simulink model "Praktikum11Gruppe09"  (R2023b)
settings: Solver=VariableStepAuto  StartTime=0.0  StopTime=0.05  RelTol=1e-3
model workspace (MAT data in the model file):
  CodeRate = 0.75
  M = 16
  PunctureVector = [1; 1; 0; 1; 0; 1]
  TracebackDepth = 48
  Trelli.numInputSymbols = 2
  Trelli.numOutputSymbols = 4
  Trelli.numStates = 64
  Trelli.nextStates = [0  32; 0  32; 1  33; 1  33; 2  34; 2  34; 3  35; 3  35; 4  36; 4  36; 5  37; 5  37; 6  38; 6  38; 7  39; 7  39; 8  40; 8  40; 9  41; 9  41; 10  42; 10  42; 11  43; 11  43; 12  44; 12  44; 13  45; 13  45; 14  46; 14  46; 15  47; 15  47; 16  48; 16  48; 17  49; 17  49; 18  50; 18  50; 19  51; 19  51; 20  52; 20  52; 21  53; 21  53; 22  54; 22  54; 23  55; 23  55; 24  56; 24  56; 25  57; 25  57; 26  58; 26  58; 27  59; 27  59; 28  60; 28  60; 29  61; 29  61; 30  62; 30  62; 31  63; 31  63]
  Trelli.outputs = [0  3; 3  0; 1  2; 2  1; 0  3; 3  0; 1  2; 2  1; 3  0; 0  3; 2  1; 1  2; 3  0; 0  3; 2  1; 1  2; 3  0; 0  3; 2  1; 1  2; 3  0; 0  3; 2  1; 1  2; 0  3; 3  0; 1  2; 2  1; 0  3; 3  0; 1  2; 2  1; 2  1; 1  2; 3  0; 0  3; 2  1; 1  2; 3  0; 0  3; 1  2; 2  1; 0  3; 3  0; 1  2; 2  1; 0  3; 3  0; 1  2; 2  1; 0  3; 3  0; 1  2; 2  1; 0  3; 3  0; 2  1; 1  2; 3  0; 0  3; 2  1; 1  2; 3  0; 0  3]
  Ts = 5e-08
undefined symbols (not defined in the file): doppler, get, gray, hot, j, magnitude
libraries: dspxfrm3 x6, dspstat3 x5, dspsigops x5, dspobslib x4, commrflib2 x3, commcnvcod2 x3, commdigbbndam3 x3, dspindex x3, commchan3 x2, commrandsrc3 x2, dspquant2 x2, commsink2 x2
settings Model: Creator=suttarar@hu-berlin.de  LastModifiedBy=suttarar@hu-berlin.de

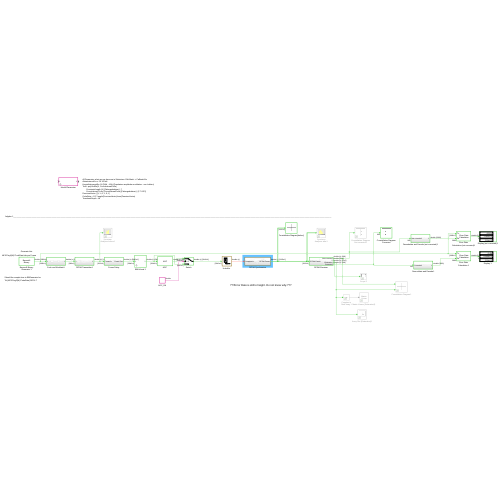
[thumbnail: Simulink's stored preview of the top-level diagram]
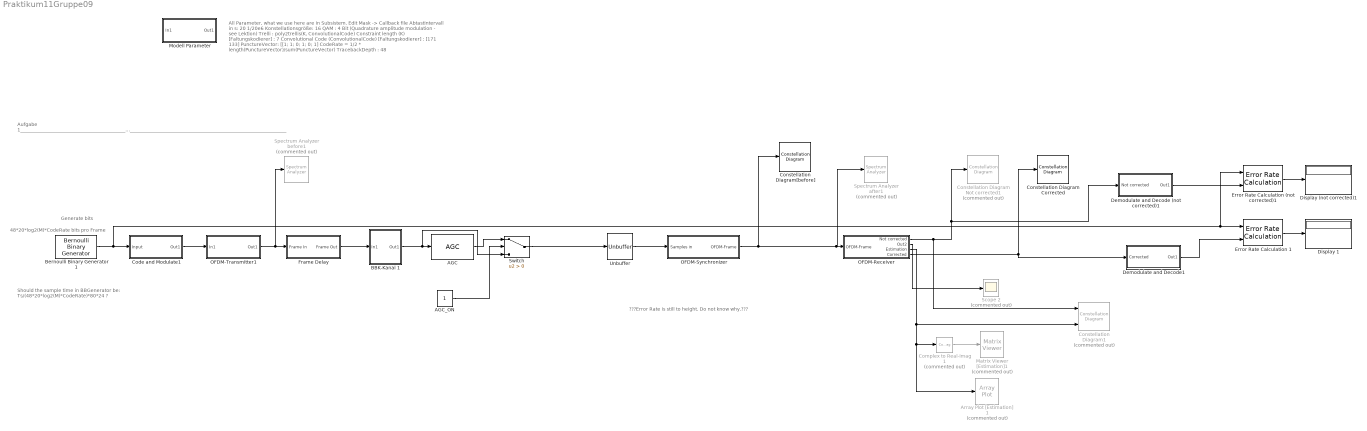
== system Praktikum11Gruppe09 ==
  note: ???Error Rate is still to height. Do not know why.???
  note: Aufgabe 1______________________________________________________________________________________________________________________________________________________________________________________________________________________________________________________________________________________________________________
  note: Should the sample time in BBGenerator be:
      | Ts/(48*20*log2(M)*CodeRate)*80*24 ?
  note: All Parameter, what we use here are in Subsistem. Edit Mask -> Callback file
      | Abtastintervall in s: 20 1/20e6
      | Konstellationsgröße: 16 QAM : 4 Bit (Quadrature amplitude modulation - see Lektion)
      | Trelli : poly2trellis(K, ConvolutionalCode)
      | Constraint length (K) [Faltungskodierer] : 7
      | Convolutional Code (ConvolutionalCode) [Faltungskodierer] : [171 133]
      | PunctureVector: [[1; 1; 0; 1; 0; 1]
      | CodeRate = 1/2 * length(PunctureVector)/sum(PunctureVector)
      | TracebackDepth : 48
  note: 48*20*log2(M)*CodeRate bits pro Frame
  note: Generate bits
  "AGC " : commrfcorlib/AGC  LegacyMode=off  DetectorMethod=Rectifier  LoopMethod=Linear  UpdatePeriod=100  StepSize=0.1  AdaptationStepSize=0.01  DesiredOutputPower=1  AveragingLength=16  MaximumGain=30  MaxPowerGain=10  GainOutputPort=off  InputPowerOutputPort=off  SimulateUsing=Interpreted execution
  AGC_ON : Constant
  Array Plot [Estimation]1 : ArrayPlot  Commented=on  WindowPosition=[886.000000,184.000000,800.000000,500.000000,]  ScopeFrameLocation=window  PlotAsMagnitudePhase=on  YLimits=[-0.4803 1.494]
  BBK-Kanal 1 : Subsystem  mask{MaxDoppler=20, PathDelays=[0 2 5].*Ts, PathGains=[0 -16 -24], EnableMultipath=1, PathLoss=0, FrequencyOffset=50000, PhaseOffset=0, SNR=25}
      mask prompts: MaxDoppler "Dopplerverschiebung"; PathDelays "Pfadverzoergerungen"; PathGains "Pfadverstaerkungen"; EnableMultipath "SwitchBlock"; PathLoss "Pfadverlust"; FrequencyOffset "Frequenzverschiebung"; PhaseOffset "Phasenverschiebung"; SNR "AWG-Rauschen"
  Bernoulli Binary Generator 1 : commrandsrc3/Bernoulli Binary Generator  ProbabilityOfZero=0.5  SeedSource=Auto  Seed=0  SampleTime=Ts/(48*20*log2(M)*CodeRate)*80*24  SamplesPerFrame=48*20*log2(M)*CodeRate  OutputDataType=double  SimulateUsing=Interpreted execution
  Code and Modulate1 : Subsystem
  Complex to Real-Imag 1 : ComplexToRealImag  Commented=on  Output=Real
  Constellation Diagram Corrected : ConstellationDiagram  WindowPosition=[869.000000,188.000000,600.000000,600.000000,]  ScopeFrameLocation=window  SymbolsToDisplaySource=Property  SymbolsToDisplay=500  ReferenceConstellation="[0.70711+0.70711i        -0.70711+0.70711i        -0.70711-0.70711i         0.70711-0.70711i]"  XLimits=[-1.71,1.66]  YLimits=[-1.67,1.51]  ShowLegend=on
  Constellation Diagram Not corrected1 : ConstellationDiagram  Commented=on  WindowPosition=[922.000000,306.000000,600.000000,600.000000,]  ScopeFrameLocation=window  ReferenceConstellation="[0.70711+0.70711i        -0.70711+0.70711i        -0.70711-0.70711i         0.70711-0.70711i]"  XLimits=[-1.55,1.51]  YLimits=[-1.43,1.46]  ShowLegend=on
  Constellation Diagram1 : ConstellationDiagram  Commented=on  NumInputPorts=2  WindowPosition=[1234.000000,143.000000,600.000000,600.000000,]  ScopeFrameLocation=window  ReferenceConstellation="{[0.70711+0.70711i        -0.70711+0.70711i        -0.70711-0.70711i         0.70711-0.70711i][0.70711+0.70711i        -0.70711+0.70711i        -0.70711-0.70711i         0.70711-0.70711i]}"  XLimits=[-1.55,1.51]  YLimits=[-1.43,1.46]  ShowLegend=on
  Constellation Diagram[before] : ConstellationDiagram  WindowPosition=[219.000000,183.000000,600.000000,600.000000,]  ScopeFrameLocation=window  SymbolsToDisplaySource=Property  SymbolsToDisplay=500  ReferenceConstellation="[0.70711+0.70711i        -0.70711+0.70711i        -0.70711-0.70711i         0.70711-0.70711i]"  XLimits=[-1.71,1.66]  YLimits=[-1.67,1.51]  ShowLegend=on
  Demodulate and Decode (not corrected)1 : Subsystem
  Demodulate and Decode1 : Subsystem
  Display (not corrected)1 : Display
  Display 1 : Display
  Error Rate Calculation (not corrected)1 : commsink2/Error Rate Calculation  N=TracebackDepth  st_delay=48*20*log2(M)*CodeRate  cp_mode=Entire frame  subframe=[]  PMode=Port  WsName=ErrorVec  RsMode2=off  stop=off  numErr=100  maxBits=1e6
  Error Rate Calculation 1 : commsink2/Error Rate Calculation  N=TracebackDepth+2880  st_delay=0  cp_mode=Entire frame  subframe=[]  PMode=Port  WsName=ErrorVec  RsMode2=off  stop=off  numErr=100  maxBits=1e6
  Frame Delay : Subsystem
  Matrix Viewer [Estimation]1 : dspobslib/Matrix Viewer  Commented=on  ImageParams=off  CMapStr=gray(256)  AxisColorbar=on  AxisParams=off  AxisOrigin=Upper left corner  AxisTickMode=Auto  XTickRange=[0 1]  YTickRange=[0 1]  XLabel=X-axis  YLabel=Y-axis  ZLabel=Z-axis  FigPos=get(0,'defaultfigureposition')  AxisZoom=off
      settings: YMin=0.99546  YMax=1.0044
  Modell Parameter : Subsystem  mask{Ts=1/20e6, M=16, Trelli=poly2trellis(7, [171 133]), PunctureVector=[1; 1; 0; 1; 0; 1], CodeRate=0.75, TracebackDepth=48}
      mask prompts: Ts "Abtastintervall in s"; M "Konstellationsgröße"
  "OFDM-Receiver " : Subsystem
  OFDM-Synchronizer : Subsystem
  OFDM-Transmitter1 : Subsystem
  Scope 2 : Scope  Commented=on
  Spectrum Analyzer after1 : SpectrumAnalyzer  Commented=on  WindowPosition=[940.000000,172.000000,800.000000,500.000000,]  Visible=on  ScopeFrameLocation=window  Span=20000000  StartFrequency=-10000000  StopFrequency=10000000  YLimits=[-28.40563685,17.66109951]
  Spectrum Analyzer before1 : SpectrumAnalyzer  Commented=on  WindowPosition=[6.000000,502.000000,800.000000,500.000000,]  ScopeFrameLocation=window  Span=20000000  StartFrequency=-10000000  StopFrequency=10000000  YLimits=[-48.78355479,20.07673212]
  "Switch " : Switch  Criteria=u2 > Threshold  SaturateOnIntegerOverflow=off  InputSameDT=off
  "Unbuffer " : Unbuffer
  wires:
  "OFDM-Receiver "/1(Not corrected) -> Constellation Diagram1/1, Demodulate and Decode (not corrected)1/1(Not corrected), Constellation Diagram Not corrected1/1
  Code and Modulate1/1(Out1) -> OFDM-Transmitter1/1(In1)
  Complex to Real-Imag 1/1 -> Matrix Viewer [Estimation]1/1
  "OFDM-Receiver "/2(Out2) -> Scope 2/1
  "OFDM-Receiver "/4(Corrected) -> Demodulate and Decode1/1(Corrected), Constellation Diagram Corrected/1
  Error Rate Calculation 1/1 -> Display 1/1
  Error Rate Calculation (not corrected)1/1 -> Display (not corrected)1/1
  Demodulate and Decode (not corrected)1/1(Out1) -> Error Rate Calculation (not corrected)1/2
  OFDM-Transmitter1/1(Out1) -> Spectrum Analyzer before1/1, Frame Delay/1(Frame In)
  Demodulate and Decode1/1(Out1) -> Error Rate Calculation 1/2
  Bernoulli Binary Generator 1/1 -> Error Rate Calculation (not corrected)1/1, Error Rate Calculation 1/1, Code and Modulate1/1(Input)
  "OFDM-Receiver "/3(Estimation) -> Constellation Diagram1/2, Array Plot [Estimation]1/1, Complex to Real-Imag 1/1
  "Unbuffer "/1 -> OFDM-Synchronizer/1(Samples in)
  BBK-Kanal 1/1(Out1) -> "Switch "/3, "AGC "/1
  Frame Delay/1(Frame Out) -> BBK-Kanal 1/1(In1)
  "Switch "/1 -> "Unbuffer "/1
  "AGC "/1 -> "Switch "/1
  AGC_ON/1 -> "Switch "/2
  OFDM-Synchronizer/1(OFDM-Frame) -> Spectrum Analyzer after1/1, "OFDM-Receiver "/1(OFDM-Frame), Constellation Diagram[before]/1

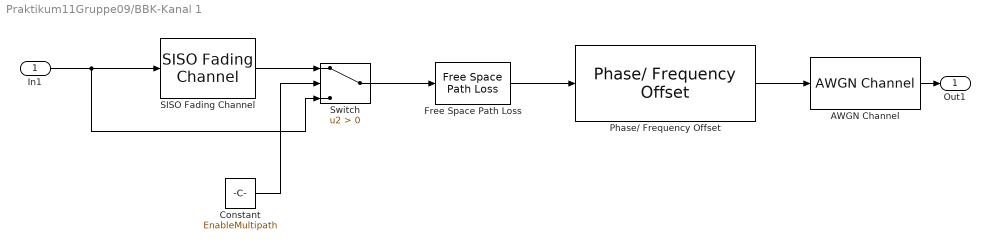
== system Praktikum11Gruppe09/BBK-Kanal 1 ==
  In1 : Inport
  AWGN Channel : commchan3/AWGN Channel  LegacyMode=off  NoiseMethod="Signal to noise ratio  (SNR)"  noiseMode="Signal to noise ratio  (SNR)"  EbNo=10  EsNo=10  SNR=SNR  BitsPerSymbol=1  SignalPower=1  SamplesPerSymbol=1  SymbolPeriod=1  VarianceSource=Parameter  Variance=1  RandomStream=Global stream  Seed=67  SimulateUsing=Code generation
  Constant : Constant  Value=EnableMultipath
  Free Space Path Loss : commrflib2/Free Space Path Loss  mode=Decibels  dB=PathLoss  d=0.100  fc=1920
  Phase/ Frequency Offset : commrflib2/Phase// Frequency Offset  phaseOffset=PhaseOffset  freqPort=off  freqOffset=FrequencyOffset
      settings: LibrarySourceBlock=|
      | commrfcorlib/Phase//
      | Frequency
      | Offset
  SISO Fading Channel : commchan3/SISO Fading Channel  InheritSampleRate=on  SampleRate=1  PathDelays=PathDelays  AveragePathGains=PathGains  NormalizePathGains=on  FadingDistribution=Rayleigh  KFactor=3  DirectPathDopplerShift=0  DirectPathInitialPhase=0  MaximumDopplerShift=MaxDoppler  DopplerSpectrum=doppler('Jakes')  RandomStream=mt19937ar with seed  Seed=73  PathGainsOutputPort=off  ChannelFilterDelayOutputPort=off  SimulateUsing=Interpreted execution  Visualization=Off  PathsForDopplerDisplay=1  SamplesToDisplay=25%
  Switch : Switch  Criteria=u2 > Threshold  SaturateOnIntegerOverflow=off  InputSameDT=off
  Out1 : Outport
  wires:
  Phase/ Frequency Offset/1 -> AWGN Channel/1
  Free Space Path Loss/1 -> Phase/ Frequency Offset/1
  AWGN Channel/1 -> Out1/1
  Switch/1 -> Free Space Path Loss/1
  SISO Fading Channel/1 -> Switch/1
  In1/1 -> Switch/3, SISO Fading Channel/1
  Constant/1 -> Switch/2

== system Praktikum11Gruppe09/Code and Modulate1 ==
  note: Modulation
  note: Faltungscodierer
  Input : Inport
  "Convolutional Encoder " : commcnvcod2/Convolutional Encoder  trellis=Trelli  opMode=Continuous  DelayedResetAction=off  hasIniStPort=off  hasFinStPort=off  usePuncVector=on  punctureVector=PunctureVector  reset=Unused parameter value
  "Rectangular QAM Modulator Baseband " : commdigbbndam3/Rectangular QAM Modulator Baseband  M=M  InType=Bit  Enc=Gray  Mapping=[0:15]  PowType=Average Power  MinDist=2  AvgPow=1  PeakPow=1  Ph=0  outDtype=double  outWordLen=16  outUDDataType=sfix(16)  outFracLenMode=Best precision  outFracLen=15  outDataTypeStr=double  outLastDataTypeStr=double
  Out1 : Outport
  wires:
  "Convolutional Encoder "/1 -> "Rectangular QAM Modulator Baseband "/1
  "Rectangular QAM Modulator Baseband "/1 -> Out1/1
  Input/1 -> "Convolutional Encoder "/1

== system Praktikum11Gruppe09/Demodulate and Decode (not corrected)1 ==
  Not corrected : Inport
  "Data Type Conversion " : DataTypeConversion  SaturateOnIntegerOverflow=off  RndMeth=Floor
  "Gain " : Gain  Gain=-1
  "Rectangular QAM Demodulator Baseband " : commdigbbndam3/Rectangular QAM Demodulator Baseband  M=M  OutType=Bit  DecType=Approximate log-likelihood ratio  VarSource=Dialog  Variance=1  Dec=Gray  Mapping=[0:15]  PowType=Average Power  MinDist=2  AvgPow=1  PeakPow=1  Ph=0  outDtype1=Inherit via internal rule  outDtype2=Inherit via internal rule  derotateFactorWordLen=16  derotateFactorDataTypeStr=Inherit: Same word length as input  derotateFactorLastDataTypeStr=Inherit: Same word length as input  denormFactorWordLen=16  denormFactorDataTypeStr=Inherit: Same word length as input  denormFactorLastDataTypeStr=Inherit: Same word length as input  prodOutWordLen=32  prodOutOverflowMode=Wrap  prodOutRoundingMode=Floor  prodOutOvFlMode=off  prodOutOvFlModeLastStrValue=off  sumWordLen=32
  "Uniform Encoder " : dspquant2/Uniform Encoder  peak=1  bits=4  otype=Unsigned integer
  "Viterbi Decoder " : commcnvcod2/Viterbi Decoder  trellis=Trelli  isPunctured=on  punctureVector=PunctureVector  erasures=off  dectype=Soft decision  nsdecb=4  runSigValErrCheck=off  tbdepth=TracebackDepth  opmode=Continuous  reset=off  delayedResetAction=off  smWordLength=16  outDataType=double
  Out1 : Outport
  wires:
  "Uniform Encoder "/1 -> "Data Type Conversion "/1
  "Gain "/1 -> "Uniform Encoder "/1
  "Data Type Conversion "/1 -> "Viterbi Decoder "/1
  "Rectangular QAM Demodulator Baseband "/1 -> "Gain "/1
  Not corrected/1 -> "Rectangular QAM Demodulator Baseband "/1
  "Viterbi Decoder "/1 -> Out1/1

== system Praktikum11Gruppe09/Demodulate and Decode1 ==
  Corrected : Inport
  "Data Type Conversion " : DataTypeConversion  SaturateOnIntegerOverflow=off  RndMeth=Floor
  "Gain " : Gain  Gain=-1
  "Rectangular QAM Demodulator Baseband " : commdigbbndam3/Rectangular QAM Demodulator Baseband  M=M  OutType=Bit  DecType=Approximate log-likelihood ratio  VarSource=Dialog  Variance=1  Dec=Gray  Mapping=[0:15]  PowType=Average Power  MinDist=2  AvgPow=1  PeakPow=1  Ph=0  outDtype1=Inherit via internal rule  outDtype2=Inherit via internal rule  derotateFactorWordLen=16  derotateFactorDataTypeStr=Inherit: Same word length as input  derotateFactorLastDataTypeStr=Inherit: Same word length as input  denormFactorWordLen=16  denormFactorDataTypeStr=Inherit: Same word length as input  denormFactorLastDataTypeStr=Inherit: Same word length as input  prodOutWordLen=32  prodOutOverflowMode=Wrap  prodOutRoundingMode=Floor  prodOutOvFlMode=off  prodOutOvFlModeLastStrValue=off  sumWordLen=32
  "Uniform Encoder " : dspquant2/Uniform Encoder  peak=1  bits=4  otype=Unsigned integer
  "Viterbi Decoder " : commcnvcod2/Viterbi Decoder  trellis=Trelli  isPunctured=on  punctureVector=PunctureVector  erasures=off  dectype=Soft decision  nsdecb=4  runSigValErrCheck=off  tbdepth=TracebackDepth  opmode=Continuous  reset=off  delayedResetAction=off  smWordLength=16  outDataType=double
  Out1 : Outport
  wires:
  "Uniform Encoder "/1 -> "Data Type Conversion "/1
  "Gain "/1 -> "Uniform Encoder "/1
  "Data Type Conversion "/1 -> "Viterbi Decoder "/1
  "Rectangular QAM Demodulator Baseband "/1 -> "Gain "/1
  Corrected/1 -> "Rectangular QAM Demodulator Baseband "/1
  "Viterbi Decoder "/1 -> Out1/1

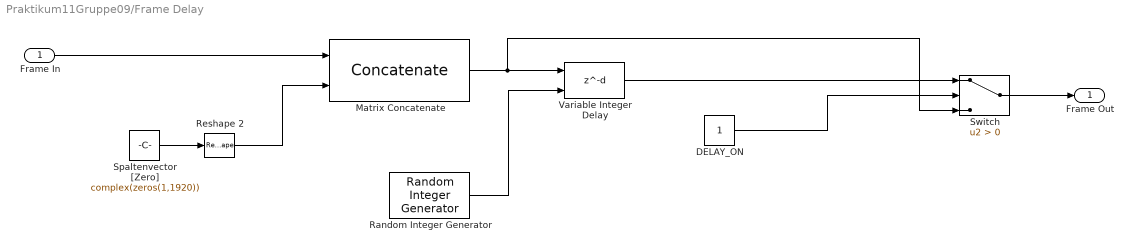
== system Praktikum11Gruppe09/Frame Delay ==
  Frame In : Inport
  DELAY_ON : Constant
  "Matrix Concatenate " : Concatenate  Mode=Multidimensional array
  "Random Integer Generator " : commrandsrc3/Random Integer Generator  SetSize=1920  SeedSource=Auto  Seed=0  SampleTime=Ts*80*24  SamplesPerFrame=1  OutputDataType=double  SimulateUsing=Interpreted execution
  Reshape 2 : Reshape  OutputDimensionality=Column vector (2-D)
  Spaltenvector [Zero] : Constant  Value=complex(zeros(1,1920))  VectorParams1D=off
  "Switch " : Switch  Criteria=u2 > Threshold  SaturateOnIntegerOverflow=off  InputSameDT=off
  "Variable Integer Delay " : Delay  DelayLengthSource=Input port  DelayLengthUpperLimit=1920  InputProcessing=Columns as channels (frame based)
      settings: InputPortMap=u0,p1
  Frame Out : Outport
  wires:
  Frame In/1 -> "Matrix Concatenate "/1
  Spaltenvector [Zero]/1 -> Reshape 2/1
  Reshape 2/1 -> "Matrix Concatenate "/2
  "Matrix Concatenate "/1 -> "Switch "/3, "Variable Integer Delay "/1
  "Random Integer Generator "/1 -> "Variable Integer Delay "/2
  "Variable Integer Delay "/1 -> "Switch "/1
  DELAY_ON/1 -> "Switch "/2
  "Switch "/1 -> Frame Out/1

== system Praktikum11Gruppe09/Modell Parameter ==
  In1 : Inport
  Out1 : Outport
  wires:
  In1/1 -> Out1/1

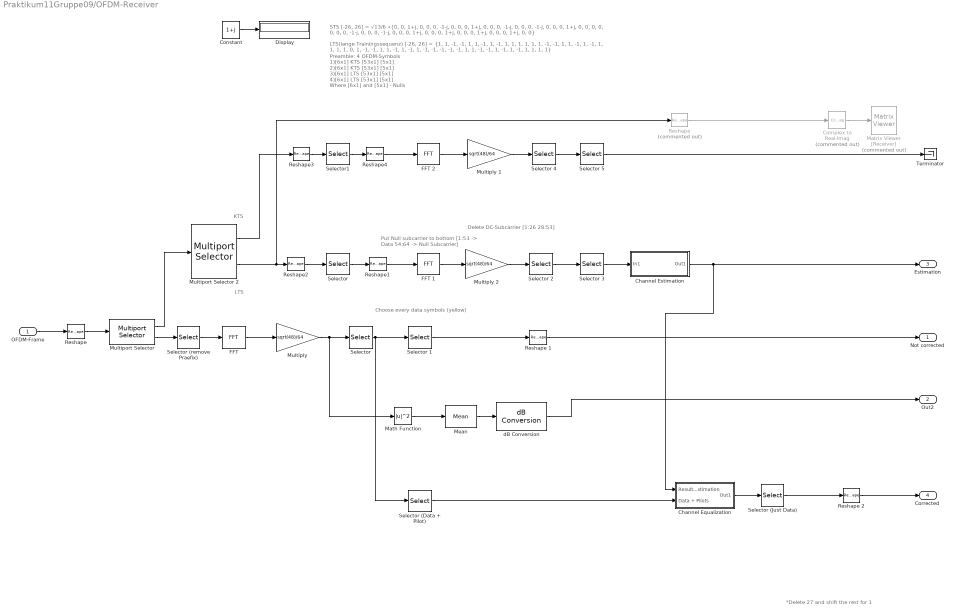
== system Praktikum11Gruppe09/OFDM-Receiver  ==
  note: *Delete 27 and shift the rest for 1
  note: Delete DC-Subcarrier [1:26 28:53]
  note: Put Null subcarrier to bottom
      | [1:53 -> Data 54:64 -> Null Subcarrier]
  note: LTS
  note: KTS
  note: Choose every data symbols (yellow)
  note: LTS(lange Trainingssequenz) [-26, 26] = {1, 1, -1, -1, 1, 1, -1, 1, -1, 1, 1, 1, 1, 1, 1, -1, -1, 1, 1, -1, 1, -1, 1, 1, 1, 1, 0, 1, -1, -1, 1, 1, -1, 1, -1, 1, -1, -1, -1, -1, -1, 1, 1, -1, -1, 1, -1, 1, -1, 1, 1, 1, 1}
  note: Preamble: 4 OFDM-Symbols
      | 1)[6x1] KTS [53x1] [5x1]
      | 2)[6x1] KTS [53x1] [5x1]
      | 3)[6x1] LTS [53x1] [5x1]
      | 4)[6x1] LTS [53x1] [5x1]
      |
      | Where [6x1] and [5x1] - Nulls
  note: STS [-26, 26] = √13/6 ∙{0, 0, 1+j, 0, 0, 0, -1-j, 0, 0, 0, 1+j, 0, 0, 0, -1-j, 0, 0, 0, -1-j, 0, 0, 0, 1+j, 0, 0, 0, 0, 0, 0, 0, -1-j, 0, 0, 0, -1-j, 0, 0, 0, 1+j, 0, 0, 0, 1+j, 0, 0, 0, 1+j, 0, 0, 0, 1+j, 0, 0}
  OFDM-Frame : Inport
  Channel Equalization : Subsystem
  Channel Estimation : Subsystem
  "Complex to Real-Imag " : ComplexToRealImag  Commented=on  Output=Real
  Constant : Constant  Value=1+j
  Display : Display
  "FFT " : dspxfrm3/FFT  FFTImplementation=Auto  CompMethod=Table lookup  TableOpt=NEW  TableOptActive=Speed  BitRevOrder=off  Normalize=off  InheritFFTLength=on  FFTLength=64  WrapInput=on  roundingMode=Floor  overflowMode=off  firstCoeffDataTypeStr=Inherit: Same word length as input  firstCoeffLastDataTypeStr=Inherit: Same word length as input  outputMin=[]  outputMax=[]
  FFT 1 : dspxfrm3/FFT  FFTImplementation=Auto  CompMethod=Table lookup  TableOpt=NEW  TableOptActive=Speed  BitRevOrder=off  Normalize=off  InheritFFTLength=on  FFTLength=64  WrapInput=on  roundingMode=Floor  overflowMode=off  firstCoeffDataTypeStr=Inherit: Same word length as input  firstCoeffLastDataTypeStr=Inherit: Same word length as input  outputMin=[]  outputMax=[]
  FFT 2 : dspxfrm3/FFT  FFTImplementation=Auto  CompMethod=Table lookup  TableOpt=NEW  TableOptActive=Speed  BitRevOrder=off  Normalize=off  InheritFFTLength=on  FFTLength=64  WrapInput=on  roundingMode=Floor  overflowMode=off  firstCoeffDataTypeStr=Inherit: Same word length as input  firstCoeffLastDataTypeStr=Inherit: Same word length as input  outputMin=[]  outputMax=[]
  "Math Function " : Math  Operator=magnitude^2
  Matrix Viewer [Receiver] : dspobslib/Matrix Viewer  Commented=on  ImageParams=off  CMapStr=gray(256)  AxisColorbar=on  AxisParams=off  AxisOrigin=Upper left corner  AxisTickMode=Auto  XTickRange=[0 1]  YTickRange=[0 1]  XLabel=X-axis  YLabel=Y-axis  ZLabel=Z-axis  FigPos=get(0,'defaultfigureposition')  AxisZoom=off
      settings: YMin=-1.4434  YMax=1.4434
  "Mean " : dspstat3/Mean  run=off  InputProcessing=Columns as channels (frame based)  reset_popup=None  directionMode=Each row  dimension=1  roiEnable=off  roiType=Rectangles  roiPortion=Entire ROI  roiOutput=Individual statistics for each ROI  roiFlag=off  roundingMode=Floor  overflowMode=off  outputDataTypeStr=Inherit: Same as accumulator  outputMin=[]  outputMax=[]  outputLastDataTypeStr=Inherit: Same as accumulator
  "Multiply " : Gain  Gain=sqrt(48)/64
  Multiply 1 : Gain  Gain=sqrt(48)/64
  Multiply 2 : Gain  Gain=sqrt(48)/64
  "Multiport Selector " : dspindex/Multiport Selector  rowsOrCols=Columns  idxCellArray={[1:4], [5:24]}  idxErrMode=Clip Index
  Multiport Selector 2 : dspindex/Multiport Selector  rowsOrCols=Columns  idxCellArray={[1:2], [3:4]}  idxErrMode=Clip Index
  Reshape : Reshape  Commented=on  OutputDimensionality=Column vector (2-D)
  "Reshape " : Reshape  OutputDimensionality=Customize  OutputDimensions=[80,24]
  Reshape 1 : Reshape  OutputDimensions=[64,24]
  Reshape 2 : Reshape  OutputDimensions=[64,24]
  Reshape1 : Reshape  OutputDimensionality=Customize  OutputDimensions=[64,2]
  Reshape2 : Reshape  OutputDimensionality=Column vector (2-D)
  Reshape3 : Reshape  OutputDimensionality=Column vector (2-D)
  Reshape4 : Reshape  OutputDimensionality=Customize  OutputDimensions=[64,2]
  Selector : Selector  NumberOfDimensions=2  InputPortWidth=3  IndexOptions=Index vector (dialog),Select all  Indices=[33:160],1  OutputSizes=1,1
  "Selector " : Selector  NumberOfDimensions=2  InputPortWidth=3  IndexOptions=Index vector (dialog),Select all  Indices=[39:64 1:38],1  OutputSizes=1,1
  Selector (remove Praefix) : Selector  NumberOfDimensions=2  InputPortWidth=3  IndexOptions=Index vector (dialog),Select all  Indices=[17:80],1  OutputSizes=1,1
  Selector (Data + Pilot) : Selector  NumberOfDimensions=2  InputPortWidth=3  IndexOptions=Index vector (dialog),Select all  Indices=[1:26 28:53],1  OutputSizes=1,1
  Selector (Just Data) : Selector  NumberOfDimensions=2  InputPortWidth=3  IndexOptions=Index vector (dialog),Select all  Indices=[1:5 7:19 21:32 34:46 48:52],1  OutputSizes=1,1
  Selector 1 : Selector  NumberOfDimensions=2  InputPortWidth=3  IndexOptions=Index vector (dialog),Select all  Indices=[1:5 7:19 21:26 28:33 35:47 49:53],1  OutputSizes=1,1
  Selector 2 : Selector  NumberOfDimensions=2  InputPortWidth=3  IndexOptions=Index vector (dialog),Select all  Indices=[39:64 1:38],1  OutputSizes=1,1
  Selector 3 : Selector  NumberOfDimensions=2  InputPortWidth=3  IndexOptions=Index vector (dialog),Select all  Indices=[1:26 28:53],1  OutputSizes=1,1
  Selector 4 : Selector  NumberOfDimensions=2  InputPortWidth=3  IndexOptions=Index vector (dialog),Select all  Indices=[39:64 1:38],1  OutputSizes=1,1
  Selector 5 : Selector  NumberOfDimensions=2  InputPortWidth=3  IndexOptions=Index vector (dialog),Select all  Indices=[1:26 28:53],1  OutputSizes=1,1
  Selector1 : Selector  NumberOfDimensions=2  InputPortWidth=3  IndexOptions=Index vector (dialog),Select all  Indices=[33:160],1  OutputSizes=1,1
  "Terminator " : Terminator
  "dB Conversion " : dspmathops/dB Conversion  dBtype=dB  intype=Power  R=1  fuzz=off
      settings: LibrarySourceBlock=commutil2/dB Conversion
  Not corrected : Outport
  Out2 : Outport  Port=2
  Estimation : Outport  Port=3
  Corrected : Outport  Port=4
  wires:
  "Mean "/1 -> "dB Conversion "/1
  "Math Function "/1 -> "Mean "/1
  "FFT "/1 -> "Multiply "/1
  OFDM-Frame/1 -> "Reshape "/1
  "Selector "/1 -> Selector (Data + Pilot)/1, Selector 1/1
  "Reshape "/1 -> "Multiport Selector "/1
  "Multiport Selector "/2 -> Selector (remove Praefix)/1
  "Multiport Selector "/1 -> Multiport Selector 2/1
  "dB Conversion "/1 -> Out2/1
  Selector 1/1 -> Reshape 1/1
  Reshape 1/1 -> Not corrected/1
  "Multiply "/1 -> "Math Function "/1, "Selector "/1
  Channel Estimation/1(Out1) -> Channel Equalization/1(Result from Channel Estimation), Estimation/1
  Selector 2/1 -> Selector 3/1
  Multiply 2/1 -> Selector 2/1
  FFT 1/1 -> Multiply 2/1
  Selector 3/1 -> Channel Estimation/1(In1)
  "Complex to Real-Imag "/1 -> Matrix Viewer [Receiver]/1
  Selector (Data + Pilot)/1 -> Channel Equalization/2(Data + Pilots)
  Channel Equalization/1(Out1) -> Selector (Just Data)/1
  Selector (Just Data)/1 -> Reshape 2/1
  Reshape 2/1 -> Corrected/1
  Selector (remove Praefix)/1 -> "FFT "/1
  Multiport Selector 2/2 -> Reshape/1, Reshape2/1
  Multiport Selector 2/1 -> Reshape3/1
  Reshape/1 -> "Complex to Real-Imag "/1
  Selector/1 -> Reshape1/1
  Reshape1/1 -> FFT 1/1
  Reshape2/1 -> Selector/1
  Constant/1 -> Display/1
  Reshape3/1 -> Selector1/1
  Selector1/1 -> Reshape4/1
  Reshape4/1 -> FFT 2/1
  FFT 2/1 -> Multiply 1/1
  Multiply 1/1 -> Selector 4/1
  Selector 4/1 -> Selector 5/1
  Selector 5/1 -> "Terminator "/1

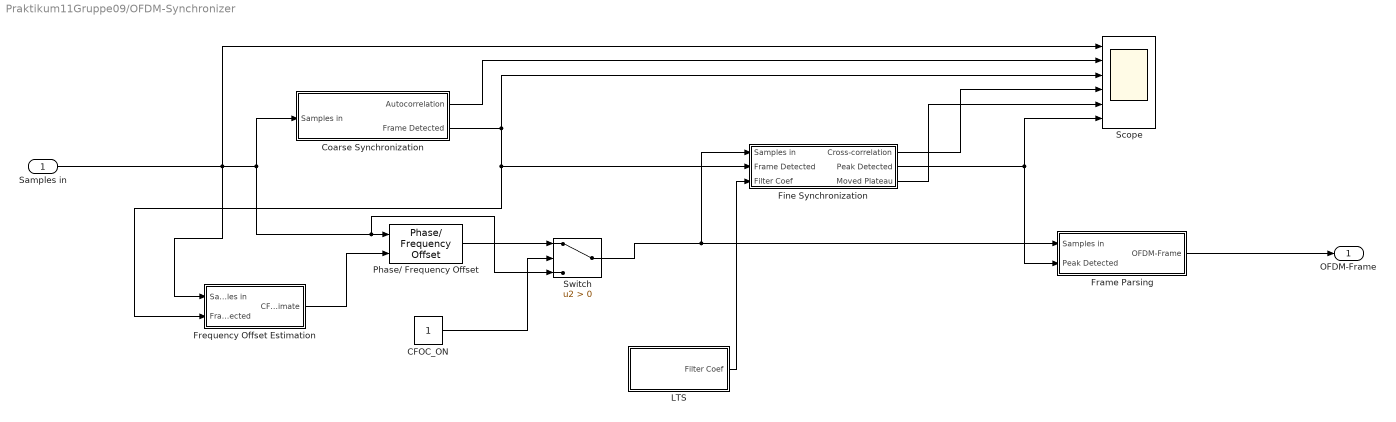
== system Praktikum11Gruppe09/OFDM-Synchronizer ==
  Samples in : Inport
  CFOC_ON : Constant
  Coarse Synchronization : Subsystem
  Fine Synchronization : Subsystem
  Frame Parsing : Subsystem
  Frequency Offset Estimation : Subsystem
  LTS : Subsystem
  Phase/ Frequency Offset : commrflib2/Phase// Frequency Offset  phaseOffset=0  freqPort=on  freqOffset=0
  "Scope " : Scope  NumInputPorts=6
  "Switch " : Switch  Criteria=u2 > Threshold  SaturateOnIntegerOverflow=off  InputSameDT=off
  OFDM-Frame : Outport
  wires:
  Fine Synchronization/2(Peak Detected) -> Frame Parsing/2(Peak Detected), "Scope "/6
  Samples in/1 -> Frequency Offset Estimation/1(Samples in), "Switch "/3, Phase/ Frequency Offset/1, Coarse Synchronization/1(Samples in), "Scope "/1
  Coarse Synchronization/2(Frame Detected) -> Frequency Offset Estimation/2(Frame Detected), Fine Synchronization/2(Frame Detected), "Scope "/3
  LTS/1(Filter Coef) -> Fine Synchronization/3(Filter Coef)
  Coarse Synchronization/1(Autocorrelation) -> "Scope "/2
  Fine Synchronization/1(Cross-correlation) -> "Scope "/4
  Fine Synchronization/3(Moved Plateau) -> "Scope "/5
  Frame Parsing/1(OFDM-Frame) -> OFDM-Frame/1
  Frequency Offset Estimation/1(CFO Estimate) -> Phase/ Frequency Offset/2
  Phase/ Frequency Offset/1 -> "Switch "/1
  "Switch "/1 -> Fine Synchronization/1(Samples in), Frame Parsing/1(Samples in)
  CFOC_ON/1 -> "Switch "/2

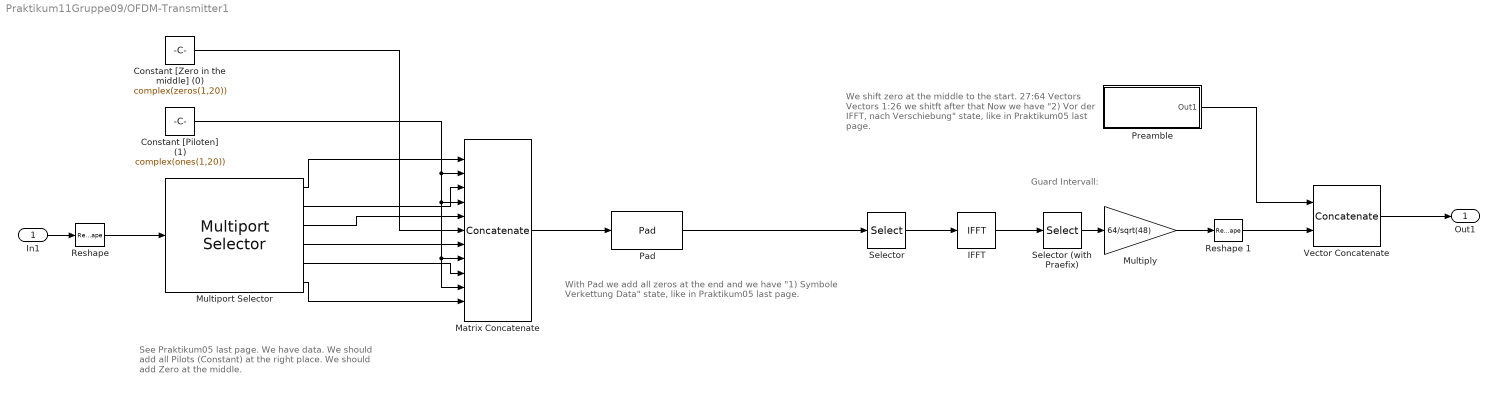
== system Praktikum11Gruppe09/OFDM-Transmitter1 ==
  note: Guard Intervall:
  note: With Pad we add all zeros at the end and we have
      | "1) Symbole Verkettung Data" state, like in Praktikum05 last page.
  note: See Praktikum05 last page. We have data.
      | We should add all Pilots (Constant) at the right place.
      | We should add Zero at the middle.
  note: We shift zero at the middle to the start.
      | 27:64 Vectors
      | Vectors 1:26 we shitft after that
      | Now we have "2) Vor der IFFT,
      | nach Verschiebung" state, like in Praktikum05 last page.
  In1 : Inport
  Constant [Piloten] (1) : Constant  Value=complex(ones(1,20))  VectorParams1D=off
  Constant [Zero in the middle] (0) : Constant  Value=complex(zeros(1,20))  VectorParams1D=off
  "IFFT " : dspxfrm3/IFFT  FFTImplementation=Auto  CompMethod=Table lookup  TableOpt=NEW  TableOptActive=Speed  BitRevOrder=off  cs_in=off  Normalize=on  InheritFFTLength=on  FFTLength=64  WrapInput=on  mode=Complex  outSamplingMode=Sample based  roundingMode=Floor  overflowMode=off  firstCoeffDataTypeStr=Inherit: Same word length as input  firstCoeffLastDataTypeStr=Inherit: Same word length as input  outputMin=[]  outputMax=[]
  "Matrix Concatenate " : Concatenate  NumInputs=11  Mode=Multidimensional array
  "Multiply " : Gain  Gain=64/sqrt(48)
  Multiport Selector : dspindex/Multiport Selector  rowsOrCols=Rows  idxCellArray={[1:5], [6:18], [19:24], [25:30], [31:43], [44:48]}  idxErrMode=Clip Index
      settings: LibrarySourceBlock=|
      | dsphdlsupportsigmgmt/Multiport
      | Selector
  "Pad " : dspsigops/Pad  padAlong=Columns  dimsToPad=1  valSrc=Specify via dialog  padVal=0  spec=Output size  padNumOutRowsSpecMethod=User-specified  numOutRows=64  padNumOutColsSpecMethod=User-specified  numOutCols=1  isVarDimsMode=off  padBeginning=0  padEnd=0  outSizeMode=User-specified  outSize=1  padSigAt=End  trunc_flag=None  roundingMode=Floor  overflowMode=off  truncOrWrapMode=Truncate  wrap_flag=None
  Preamble : Subsystem
  "Reshape " : Reshape  OutputDimensionality=Customize  OutputDimensions=[48,20]
  Reshape 1 : Reshape  OutputDimensionality=Column vector (2-D)  OutputDimensions=[64,24]
  "Selector " : Selector  NumberOfDimensions=2  InputPortWidth=3  IndexOptions=Index vector (dialog),Select all  Indices=[27:64 1:26],1  OutputSizes=1,1
  Selector (with Praefix) : Selector  NumberOfDimensions=2  InputPortWidth=3  IndexOptions=Index vector (dialog),Select all  Indices=[49:64, 1:64],1  OutputSizes=1,1
  "Vector Concatenate " : Concatenate
  Out1 : Outport
  wires:
  In1/1 -> "Reshape "/1
  "Reshape "/1 -> Multiport Selector/1
  "Pad "/1 -> "Selector "/1
  "Matrix Concatenate "/1 -> "Pad "/1
  Multiport Selector/1 -> "Matrix Concatenate "/1
  Multiport Selector/2 -> "Matrix Concatenate "/3
  Multiport Selector/3 -> "Matrix Concatenate "/5
  Multiport Selector/4 -> "Matrix Concatenate "/7
  Multiport Selector/5 -> "Matrix Concatenate "/9
  Multiport Selector/6 -> "Matrix Concatenate "/11
  Constant [Piloten] (1)/1 -> "Matrix Concatenate "/10, "Matrix Concatenate "/8, "Matrix Concatenate "/4, "Matrix Concatenate "/2
  Constant [Zero in the middle] (0)/1 -> "Matrix Concatenate "/6
  "Selector "/1 -> "IFFT "/1
  "IFFT "/1 -> Selector (with Praefix)/1
  "Multiply "/1 -> Reshape 1/1
  Reshape 1/1 -> "Vector Concatenate "/2
  "Vector Concatenate "/1 -> Out1/1
  Preamble/1(Out1) -> "Vector Concatenate "/1
  Selector (with Praefix)/1 -> "Multiply "/1

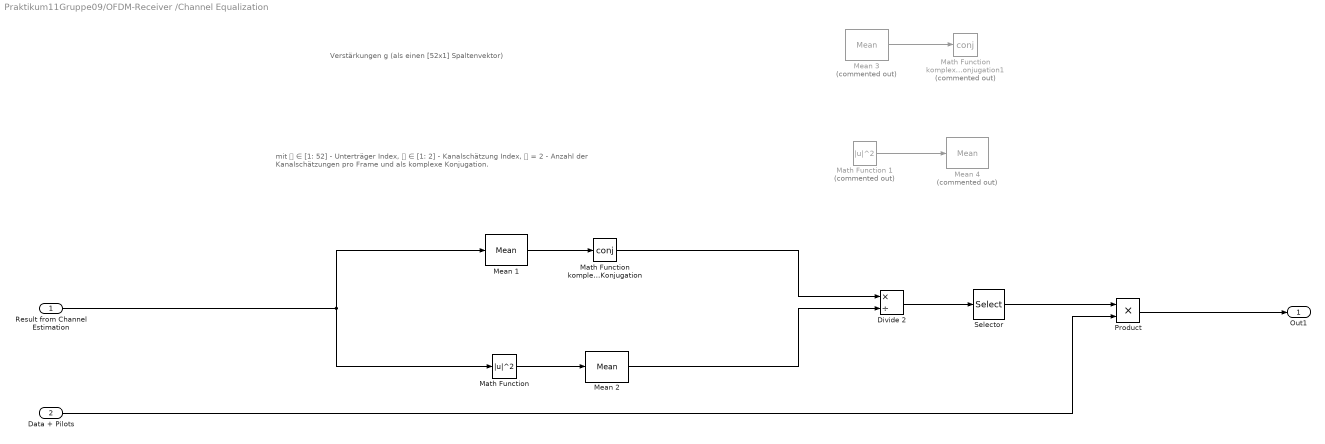
== system Praktikum11Gruppe09/OFDM-Receiver /Channel Equalization ==
  note: mit 𝑢 ∈ [1: 52] - Unterträger Index, 𝑛 ∈ [1: 2] - Kanalschätzung Index, 𝑁 = 2 - Anzahl der Kanalschätzungen pro Frame und als komplexe Konjugation.
  note: Verstärkungen g (als einen [52x1] Spaltenvektor)
  Result from Channel Estimation : Inport
  Data + Pilots : Inport  Port=2
  Divide 2 : Product  Inputs=*/
  "Math Function " : Math  Operator=magnitude^2
  Math Function 1 : Math  Commented=on  Operator=magnitude^2
  Math Function komplexe Konjugation : Math  Operator=conj  OutputSignalType=complex
  Math Function komplexe Konjugation1 : Math  Commented=on  Operator=conj  OutputSignalType=complex
  Mean 1 : dspstat3/Mean  run=off  InputProcessing=Columns as channels (frame based)  reset_popup=None  directionMode=Each row  dimension=1  roiEnable=off  roiType=Rectangles  roiPortion=Entire ROI  roiOutput=Individual statistics for each ROI  roiFlag=off  roundingMode=Floor  overflowMode=off  outputDataTypeStr=Inherit: Same as accumulator  outputMin=[]  outputMax=[]  outputLastDataTypeStr=Inherit: Same as accumulator
  Mean 2 : dspstat3/Mean  run=off  InputProcessing=Columns as channels (frame based)  reset_popup=None  directionMode=Each row  dimension=1  roiEnable=off  roiType=Rectangles  roiPortion=Entire ROI  roiOutput=Individual statistics for each ROI  roiFlag=off  roundingMode=Floor  overflowMode=off  outputDataTypeStr=Inherit: Same as accumulator  outputMin=[]  outputMax=[]  outputLastDataTypeStr=Inherit: Same as accumulator
  Mean 3 : dspstat3/Mean  Commented=on  run=off  InputProcessing=Columns as channels (frame based)  reset_popup=None  directionMode=Each row  dimension=1  roiEnable=off  roiType=Rectangles  roiPortion=Entire ROI  roiOutput=Individual statistics for each ROI  roiFlag=off  roundingMode=Floor  overflowMode=off  outputDataTypeStr=Inherit: Same as accumulator  outputMin=[]  outputMax=[]  outputLastDataTypeStr=Inherit: Same as accumulator
  Mean 4 : dspstat3/Mean  Commented=on  run=off  InputProcessing=Columns as channels (frame based)  reset_popup=None  directionMode=Each row  dimension=1  roiEnable=off  roiType=Rectangles  roiPortion=Entire ROI  roiOutput=Individual statistics for each ROI  roiFlag=off  roundingMode=Floor  overflowMode=off  outputDataTypeStr=Inherit: Same as accumulator  outputMin=[]  outputMax=[]  outputLastDataTypeStr=Inherit: Same as accumulator
  "Product " : Product
  "Selector " : Selector  NumberOfDimensions=2  InputPortWidth=3  IndexOptions=Select all,Index vector (dialog)  Indices=[1 3],ones(20,1)  OutputSizes=1,1
  Out1 : Outport
  wires:
  Result from Channel Estimation/1 -> "Math Function "/1, Mean 1/1
  Mean 1/1 -> Math Function komplexe Konjugation/1
  Math Function komplexe Konjugation/1 -> Divide 2/1
  "Math Function "/1 -> Mean 2/1
  Mean 2/1 -> Divide 2/2
  Mean 3/1 -> Math Function komplexe Konjugation1/1
  Math Function 1/1 -> Mean 4/1
  Divide 2/1 -> "Selector "/1
  Data + Pilots/1 -> "Product "/2
  "Selector "/1 -> "Product "/1
  "Product "/1 -> Out1/1

== system Praktikum11Gruppe09/OFDM-Receiver /Channel Estimation ==
  note: We should divide recieved data to transmitted data
      | *remove 0, we can't divide to 0
  note: LTS(lange Trainingssequenz) [-26, 26] = {1, 1, -1, -1, 1, 1, -1, 1, -1, 1, 1, 1, 1, 1, 1, -1, -1, 1, 1, -1, 1, -1, 1, 1, 1, 1, 0, 1, -1, -1, 1, 1, -1, 1, -1, 1, -1, -1, -1, -1, -1, 1, 1, -1, -1, 1, -1, 1, -1, 1, 1, 1, 1}
  In1 : Inport
  "Divide " : Product  Inputs=*/
  "LTS [-26, 26]" : Constant  Value=complex([1, 1, -1, -1, 1, 1, -1, 1, -1, 1, 1, 1, 1, 1, 1, -1, -1, 1, 1, -1, 1, -1, 1, 1, 1, 1, 0, 1, -1, -1, 1, 1, -1, 1, -1, 1, -1, -1, -1, -1, -1, 1, 1, -1, -1, 1, -1, 1, -1, 1, 1, 1, 1])  VectorParams1D=off
  Matrix Concatenate 2 : Concatenate  Mode=Multidimensional array  ConcatenateDimension=2
  "Reshape " : Reshape  OutputDimensionality=Column vector (2-D)
  "Selector " : Selector  NumberOfDimensions=2  InputPortWidth=3  IndexOptions=Index vector (dialog),Select all  Indices=[1:26 28:53],1  OutputSizes=1,1
  Out1 : Outport
  wires:
  "LTS [-26, 26]"/1 -> "Reshape "/1
  "Reshape "/1 -> Matrix Concatenate 2/2, Matrix Concatenate 2/1
  Matrix Concatenate 2/1 -> "Selector "/1
  "Selector "/1 -> "Divide "/2
  In1/1 -> "Divide "/1
  "Divide "/1 -> Out1/1

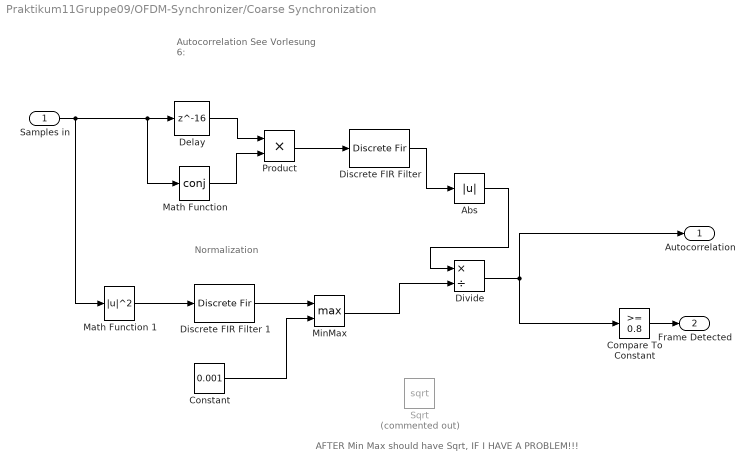
== system Praktikum11Gruppe09/OFDM-Synchronizer/Coarse Synchronization ==
  note: AFTER Min Max should have Sqrt, IF I HAVE A PROBLEM!!!
  note: Normalization
  note: Autocorrelation
      | See Vorlesung 6:
  Samples in : Inport
  "Abs " : Abs  SaturateOnIntegerOverflow=off
  "Compare To Constant " : simulink/Logic and Bit Operations/Compare To Constant  relop=>=  const=0.8  OutDataTypeStr=boolean
  "Constant " : Constant  Value=0.001
  "Delay " : Delay  DelayLength=16
  "Discrete FIR Filter " : DiscreteFir  Coefficients=ones(1,16)./16
  Discrete FIR Filter 1 : DiscreteFir  Coefficients=ones(1,16)./16
  Divide : Product  Inputs=*/
  "Math Function " : Math  Operator=conj
  Math Function 1 : Math  Operator=magnitude^2
  "MinMax " : MinMax  Function=max  Inputs=2
  "Product " : Product
  Sqrt : Sqrt  Commented=on
  Autocorrelation : Outport
  Frame Detected : Outport  Port=2
  wires:
  Samples in/1 -> "Math Function "/1, "Delay "/1, Math Function 1/1
  "Delay "/1 -> "Product "/1
  "Math Function "/1 -> "Product "/2
  "Product "/1 -> "Discrete FIR Filter "/1
  "Discrete FIR Filter "/1 -> "Abs "/1
  "Abs "/1 -> Divide/1
  "Compare To Constant "/1 -> Frame Detected/1
  Math Function 1/1 -> Discrete FIR Filter 1/1
  "Constant "/1 -> "MinMax "/2
  Discrete FIR Filter 1/1 -> "MinMax "/1
  "MinMax "/1 -> Divide/2
  Divide/1 -> Autocorrelation/1, "Compare To Constant "/1

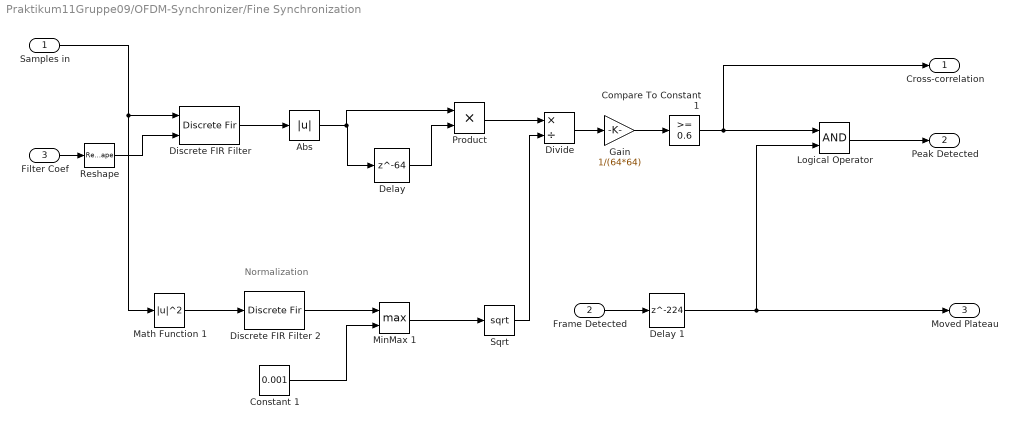
== system Praktikum11Gruppe09/OFDM-Synchronizer/Fine Synchronization ==
  note: Normalization
  Samples in : Inport
  Frame Detected : Inport  Port=2
  Filter Coef : Inport  Port=3
  "Abs " : Abs  SaturateOnIntegerOverflow=off
  Compare To Constant 1 : simulink/Logic and Bit Operations/Compare To Constant  relop=>=  const=0.6  OutDataTypeStr=boolean
  Constant 1 : Constant  Value=0.001
  "Delay " : Delay  DelayLength=64
  Delay 1 : Delay  DelayLength=224
  "Discrete FIR Filter " : DiscreteFir  CoefSource=Input port  Coefficients=16
      settings: InputPortMap=u0,u1
  Discrete FIR Filter 2 : DiscreteFir  Coefficients=ones(1,64)./64
  Divide : Product  Inputs=*/
  Gain : Gain  Gain=1/(64*64)
  "Logical Operator " : Logic  AllPortsSameDT=off  OutDataTypeStr=boolean
  Math Function 1 : Math  Operator=magnitude^2
  MinMax 1 : MinMax  Function=max  Inputs=2
  "Product " : Product
  "Reshape " : Reshape  OutputDimensionality=Row vector (2-D)
  "Sqrt " : Sqrt
  Cross-correlation : Outport
  Peak Detected : Outport  Port=2
  Moved Plateau : Outport  Port=3
  wires:
  Filter Coef/1 -> "Reshape "/1
  "Reshape "/1 -> "Discrete FIR Filter "/2
  Samples in/1 -> Math Function 1/1, "Discrete FIR Filter "/1
  "Discrete FIR Filter "/1 -> "Abs "/1
  "Abs "/1 -> "Product "/1, "Delay "/1
  "Delay "/1 -> "Product "/2
  Math Function 1/1 -> Discrete FIR Filter 2/1
  Constant 1/1 -> MinMax 1/2
  Discrete FIR Filter 2/1 -> MinMax 1/1
  Frame Detected/1 -> Delay 1/1
  "Product "/1 -> Divide/1
  MinMax 1/1 -> "Sqrt "/1
  "Sqrt "/1 -> Divide/2
  Divide/1 -> Gain/1
  Delay 1/1 -> Moved Plateau/1, "Logical Operator "/2
  Compare To Constant 1/1 -> Cross-correlation/1, "Logical Operator "/1
  "Logical Operator "/1 -> Peak Detected/1
  Gain/1 -> Compare To Constant 1/1

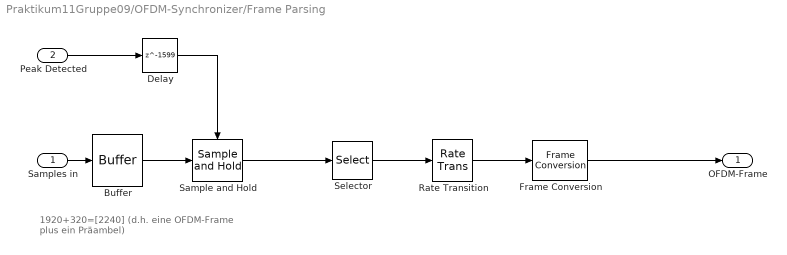
== system Praktikum11Gruppe09/OFDM-Synchronizer/Frame Parsing ==
  note: 1920+320=[2240]
      | (d.h. eine OFDM-Frame plus ein Präambel)
  Samples in : Inport
  Peak Detected : Inport  Port=2
  "Buffer " : Buffer  N=1920+320  V=2239  OutputFrames=off
  "Delay " : Delay  DelayLength=1599
  "Frame Conversion " : FrameConversion
  "Rate Transition " : RateTransition
  "Sample and Hold " : dspsigops/Sample and Hold  trig=Rising edge  initCond=0  latchinput=off
  "Selector " : Selector  NumberOfDimensions=2  InputPortWidth=3  IndexOptions=Index vector (dialog),Select all  Indices=[321:2240],[321:2240]  OutputSizes=1,1
  OFDM-Frame : Outport
  wires:
  Samples in/1 -> "Buffer "/1
  "Buffer "/1 -> "Sample and Hold "/1
  "Sample and Hold "/1 -> "Selector "/1
  Peak Detected/1 -> "Delay "/1
  "Delay "/1 -> "Sample and Hold "/Trigger
  "Selector "/1 -> "Rate Transition "/1
  "Rate Transition "/1 -> "Frame Conversion "/1
  "Frame Conversion "/1 -> OFDM-Frame/1

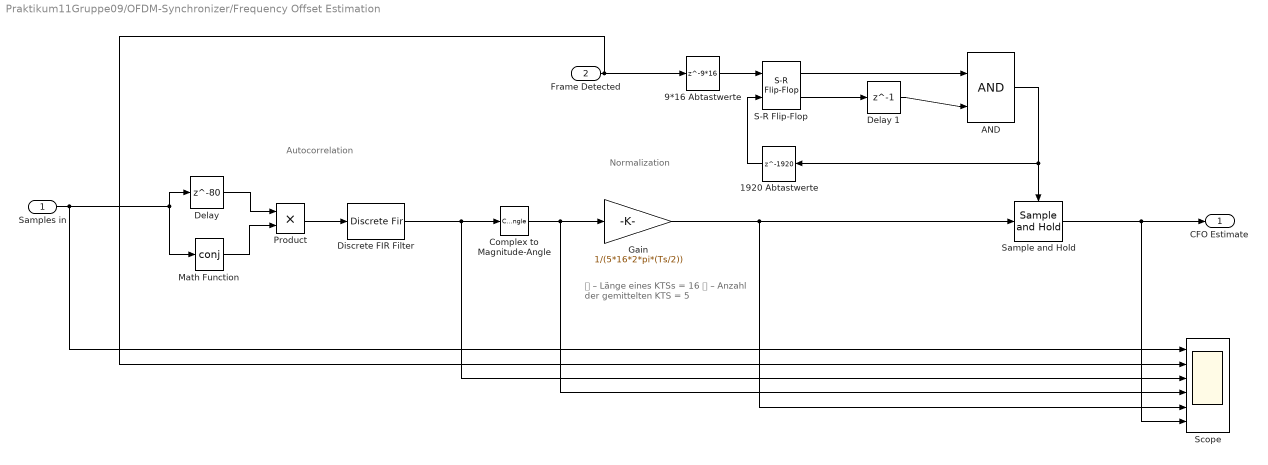
== system Praktikum11Gruppe09/OFDM-Synchronizer/Frequency Offset Estimation ==
  note: Autocorrelation
  note: 𝐿 – Länge eines KTSs = 16
      | 𝑁 – Anzahl der gemittelten KTS = 5
  note: Normalization
  Samples in : Inport
  Frame Detected : Inport  Port=2
  1920 Abtastwerte : Delay  DelayLength=1920
  "9*16 Abtastwerte " : Delay  DelayLength=9*16
  "AND " : Logic  IconShape=distinctive  AllPortsSameDT=off  OutDataTypeStr=boolean
  "Complex to Magnitude-Angle " : ComplexToMagnitudeAngle  Output=Angle
  "Delay " : Delay  DelayLength=80
  Delay 1 : Delay  DelayLength=1
  "Discrete FIR Filter " : DiscreteFir  Coefficients=ones(1,80)
  "Gain " : Gain  Gain=1/(5*16*2*pi*(Ts/2))
  "Math Function " : Math  Operator=conj
  "Product " : Product
  "S-R Flip-Flop " : simulink_extras/Flip Flops/S-R Flip-Flop  initial_condition=0
  Sample and Hold : dspsigops/Sample and Hold  trig=Rising edge  initCond=0  latchinput=off
  "Scope " : Scope  NumInputPorts=6
  CFO Estimate : Outport
  wires:
  Frame Detected/1 -> "9*16 Abtastwerte "/1, "Scope "/2
  "9*16 Abtastwerte "/1 -> "S-R Flip-Flop "/1
  1920 Abtastwerte/1 -> "S-R Flip-Flop "/2
  "Math Function "/1 -> "Product "/2
  Samples in/1 -> "Scope "/1, "Math Function "/1, "Delay "/1
  "Delay "/1 -> "Product "/1
  "Product "/1 -> "Discrete FIR Filter "/1
  "Discrete FIR Filter "/1 -> "Scope "/3, "Complex to Magnitude-Angle "/1
  "Complex to Magnitude-Angle "/1 -> "Scope "/4, "Gain "/1
  Sample and Hold/1 -> "Scope "/6, CFO Estimate/1
  "Gain "/1 -> "Scope "/5, Sample and Hold/1
  "S-R Flip-Flop "/2 -> Delay 1/1
  "S-R Flip-Flop "/1 -> "AND "/1
  Delay 1/1 -> "AND "/2
  "AND "/1 -> 1920 Abtastwerte/1, Sample and Hold/Trigger

== system Praktikum11Gruppe09/OFDM-Synchronizer/LTS ==
  "IFFT " : dspxfrm3/IFFT  FFTImplementation=Auto  CompMethod=Table lookup  TableOpt=NEW  TableOptActive=Speed  BitRevOrder=off  cs_in=off  Normalize=on  InheritFFTLength=on  FFTLength=64  WrapInput=on  mode=Complex  outSamplingMode=Sample based  roundingMode=Floor  overflowMode=off  firstCoeffDataTypeStr=Inherit: Same word length as input  firstCoeffLastDataTypeStr=Inherit: Same word length as input  outputMin=[]  outputMax=[]
  "LTS [-26, 26]" : Constant  Value=complex([1, 1, -1, -1, 1, 1, -1, 1, -1, 1, 1, 1, 1, 1, 1, -1, -1, 1, 1, -1, 1, -1, 1, 1, 1, 1, 0, 1, -1, -1, 1, 1, -1, 1, -1, 1, -1, -1, -1, -1, -1, 1, 1, -1, -1, 1, -1, 1, -1, 1, 1, 1, 1])  VectorParams1D=off
  "Multiply " : Gain  Gain=64/sqrt(48)
  "Pad " : dspsigops/Pad  padAlong=Columns  dimsToPad=1  valSrc=Specify via dialog  padVal=0  spec=Output size  padNumOutRowsSpecMethod=User-specified  numOutRows=64  padNumOutColsSpecMethod=User-specified  numOutCols=1  isVarDimsMode=off  padBeginning=0  padEnd=0  outSizeMode=User-specified  outSize=1  padSigAt=End  trunc_flag=None  roundingMode=Floor  overflowMode=off  truncOrWrapMode=Truncate  wrap_flag=None
  "Reshape " : Reshape  OutputDimensionality=Column vector (2-D)
  "Selector " : Selector  NumberOfDimensions=2  InputPortWidth=3  IndexOptions=Index vector (dialog),Select all  Indices=[27:64 1:26],1  OutputSizes=1,1
  Filter Coef : Outport
  wires:
  "LTS [-26, 26]"/1 -> "Reshape "/1
  "Reshape "/1 -> "Pad "/1
  "Pad "/1 -> "Selector "/1
  "Selector "/1 -> "IFFT "/1
  "IFFT "/1 -> "Multiply "/1
  "Multiply "/1 -> Filter Coef/1

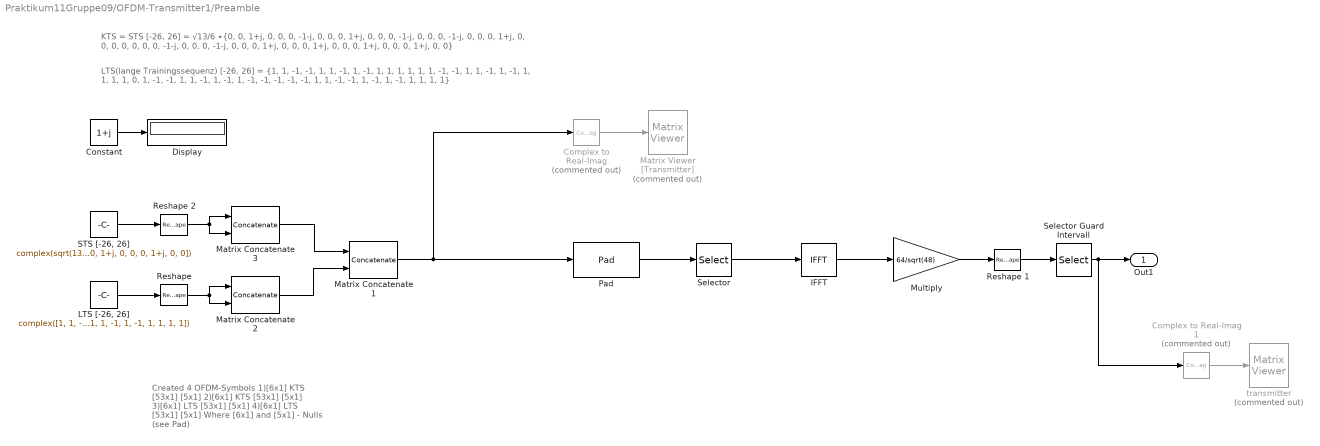
== system Praktikum11Gruppe09/OFDM-Transmitter1/Preamble ==
  note: KTS = STS [-26, 26] = √13/6 ∙{0, 0, 1+j, 0, 0, 0, -1-j, 0, 0, 0, 1+j, 0, 0, 0, -1-j, 0, 0, 0, -1-j, 0, 0, 0, 1+j, 0, 0, 0, 0, 0, 0, 0, -1-j, 0, 0, 0, -1-j, 0, 0, 0, 1+j, 0, 0, 0, 1+j, 0, 0, 0, 1+j, 0, 0, 0, 1+j, 0, 0}
  note: Created 4 OFDM-Symbols
      | 1)[6x1] KTS [53x1] [5x1]
      | 2)[6x1] KTS [53x1] [5x1]
      | 3)[6x1] LTS [53x1] [5x1]
      | 4)[6x1] LTS [53x1] [5x1]
      |
      | Where [6x1] and [5x1] - Nulls (see Pad)
  note: LTS(lange Trainingssequenz) [-26, 26] = {1, 1, -1, -1, 1, 1, -1, 1, -1, 1, 1, 1, 1, 1, 1, -1, -1, 1, 1, -1, 1, -1, 1, 1, 1, 1, 0, 1, -1, -1, 1, 1, -1, 1, -1, 1, -1, -1, -1, -1, -1, 1, 1, -1, -1, 1, -1, 1, -1, 1, 1, 1, 1}
  "Complex to Real-Imag " : ComplexToRealImag  Commented=on  Output=Real
  Complex to Real-Imag 1 : ComplexToRealImag  Commented=on  Output=Real
  Constant : Constant  Value=1+j
  Display : Display
  "IFFT " : dspxfrm3/IFFT  FFTImplementation=Auto  CompMethod=Table lookup  TableOpt=NEW  TableOptActive=Speed  BitRevOrder=off  cs_in=off  Normalize=on  InheritFFTLength=on  FFTLength=64  WrapInput=on  mode=Complex  outSamplingMode=Sample based  roundingMode=Floor  overflowMode=off  firstCoeffDataTypeStr=Inherit: Same word length as input  firstCoeffLastDataTypeStr=Inherit: Same word length as input  outputMin=[]  outputMax=[]
  "LTS [-26, 26]" : Constant  Value=complex([1, 1, -1, -1, 1, 1, -1, 1, -1, 1, 1, 1, 1, 1, 1, -1, -1, 1, 1, -1, 1, -1, 1, 1, 1, 1, 0, 1, -1, -1, 1, 1, -1, 1, -1, 1, -1, -1, -1, -1, -1, 1, 1, -1, -1, 1, -1, 1, -1, 1, 1, 1, 1])  VectorParams1D=off
  Matrix Concatenate 1 : Concatenate  Mode=Multidimensional array  ConcatenateDimension=2
  Matrix Concatenate 2 : Concatenate  Mode=Multidimensional array  ConcatenateDimension=2
  Matrix Concatenate 3 : Concatenate  Mode=Multidimensional array  ConcatenateDimension=2
  Matrix Viewer [Transmitter] : dspobslib/Matrix Viewer  Commented=on  ImageParams=off  CMapStr=hot(256)  AxisColorbar=on  AxisParams=off  AxisOrigin=Upper left corner  AxisTickMode=User-defined  XTickRange=[1 4]  YTickRange=[1 53]  XLabel=X-axis  YLabel=Y-axis  ZLabel=Z-axis  FigPos=get(0,'defaultfigureposition')  AxisZoom=off
      settings: YMin=-1  YMax=1
  "Multiply " : Gain  Gain=64/sqrt(48)
  "Pad " : dspsigops/Pad  padAlong=Columns  dimsToPad=1  valSrc=Specify via dialog  padVal=0  spec=Output size  padNumOutRowsSpecMethod=User-specified  numOutRows=64  padNumOutColsSpecMethod=User-specified  numOutCols=1  isVarDimsMode=off  padBeginning=0  padEnd=0  outSizeMode=User-specified  outSize=1  padSigAt=End  trunc_flag=None  roundingMode=Floor  overflowMode=off  truncOrWrapMode=Truncate  wrap_flag=None
  "Reshape " : Reshape  OutputDimensionality=Column vector (2-D)
  Reshape 1 : Reshape  OutputDimensionality=Column vector (2-D)  OutputDimensions=[64,24]
  Reshape 2 : Reshape  OutputDimensionality=Column vector (2-D)
  "STS [-26, 26] " : Constant  Value=complex(sqrt(13/6)*[0, 0, 1+j, 0, 0, 0, -1-j, 0, 0, 0, 1+j, 0, 0, 0, -1-j, 0, 0, 0, -1-j, 0, 0, 0, 1+j, 0, 0, 0, 0, 0, 0, 0, -1-j, 0, 0, 0, -1-j, 0, 0, 0, 1+j, 0, 0, 0, 1+j, 0, 0, 0, 1+j, 0, 0, 0, 1+j, 0, 0])  VectorParams1D=off
  "Selector " : Selector  NumberOfDimensions=2  InputPortWidth=3  IndexOptions=Index vector (dialog),Select all  Indices=[27:64 1:26],1  OutputSizes=1,1
  Selector Guard Intervall : Selector  NumberOfDimensions=2  InputPortWidth=3  IndexOptions=Index vector (dialog),Select all  Indices=[33:64, 1:128, 225:256, 129:256],1  OutputSizes=1,1
  transmitter : dspobslib/Matrix Viewer  Commented=on  ImageParams=off  CMapStr=gray(256)  AxisColorbar=on  AxisParams=off  AxisOrigin=Upper left corner  AxisTickMode=Auto  XTickRange=[0 1]  YTickRange=[0 1]  XLabel=X-axis  YLabel=Y-axis  ZLabel=Z-axis  FigPos=get(0,'defaultfigureposition')  AxisZoom=off
      settings: YMin=-1.4434  YMax=7.6499
  Out1 : Outport
  wires:
  "Pad "/1 -> "Selector "/1
  "Selector "/1 -> "IFFT "/1
  Reshape 1/1 -> Selector Guard Intervall/1
  Matrix Concatenate 1/1 -> "Pad "/1, "Complex to Real-Imag "/1
  "LTS [-26, 26]"/1 -> "Reshape "/1
  "Reshape "/1 -> Matrix Concatenate 2/2, Matrix Concatenate 2/1
  Matrix Concatenate 2/1 -> Matrix Concatenate 1/2
  "Complex to Real-Imag "/1 -> Matrix Viewer [Transmitter]/1
  "IFFT "/1 -> "Multiply "/1
  "Multiply "/1 -> Reshape 1/1
  Complex to Real-Imag 1/1 -> transmitter/1
  Selector Guard Intervall/1 -> Complex to Real-Imag 1/1, Out1/1
  "STS [-26, 26] "/1 -> Reshape 2/1
  Reshape 2/1 -> Matrix Concatenate 3/2, Matrix Concatenate 3/1
  Matrix Concatenate 3/1 -> Matrix Concatenate 1/1
  Constant/1 -> Display/1
